simulink model "Mo_hinh_dao_chieu_dong_co_1c_kich_tu_doc_lap"  (R2016a)
settings: Solver=VariableStepAuto  StartTime=0.0  StopTime=10.0  RelTol=1e-3
libraries: powerlib x14, simulink x1
settings Model: Creator=Admin  LastModifiedBy=Admin

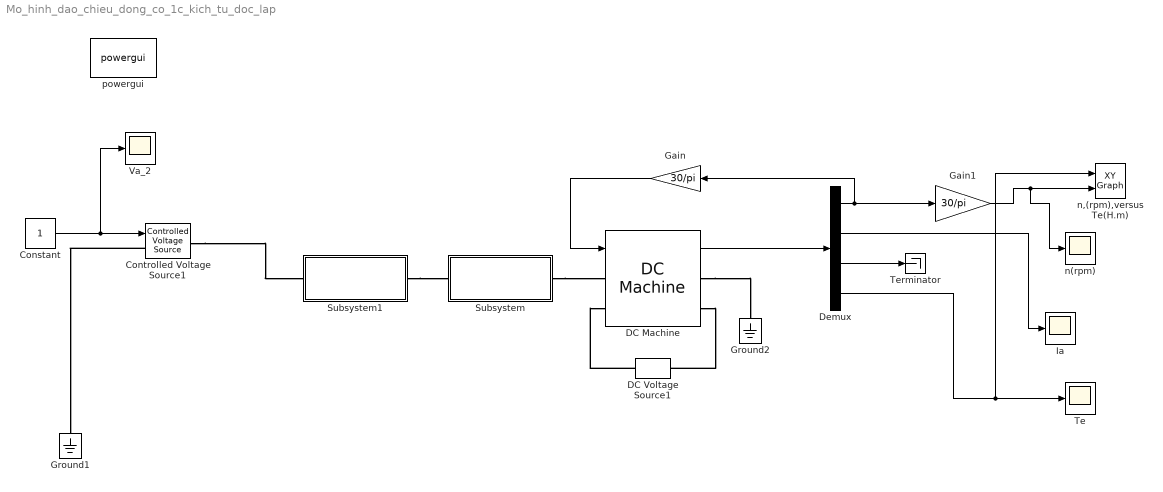
== system Mo_hinh_dao_chieu_dong_co_1c_kich_tu_doc_lap ==
  Constant : Constant
  Controlled Voltage Source1 : powerlib/Electrical Sources/Controlled Voltage Source  Initialize=on  Source_Type=AC  Amplitude=0  Phase=0  Frequency=0  Measurements=None
  DC Machine : powerlib/Machines/DC Machine  PresetModel=No  MechanicalLoad=Torque TL  FieldType=Wound  ShowDetailedParameters=on  MeasurementBus=off  RLa=[ 0.348 0.0174]  RLf=[ 0.143 0.143]  Laf=0.0174  MachineConstant=Torque constant (N.m/A)  Ke=1.8  Kt=1.8  J=1.22  Bm=0.14  Tf=2.7  w0=1  Ifinit=1  TsPowergui=0  TsBlock=-1
  DC Voltage Source1 : powerlib/Electrical Sources/DC Voltage Source  Amplitude=220  Measurements=None
  Demux : Demux
  Gain : Gain  Gain=30/pi
  Gain1 : Gain  Gain=30/pi
  Ground1 : powerlib/Elements/Ground  LConnTagsString=a
  Ground2 : powerlib/Elements/Ground  LConnTagsString=a
  "Ia " : Scope
  Subsystem : Subsystem
  Subsystem1 : Subsystem
  "Te " : Scope
  Terminator : Terminator
  "Va_2 " : Scope
  "n(rpm) " : Scope
  "n,(rpm),versus Te(H.m) " : simulink/Sinks/XY Graph  xmin=-1  xmax=1  ymin=-1  ymax=1  st=-1
  powergui : powerlib/powergui  Priority=1  SimulationMode=Continuous  SolverType=Tustin/Backward Euler (TBE)  SampleTime=50e-6  frequency=60  SPID=off  DisableSnubberDevices=off  DisableRonSwitches=off  DisableVfSwitches=off  SwTol=0  DisplayEquations=off  Interpol=off  ExternalGateDelay=off  methode=off  Ts=10  FunctionMessages=off  echomessages=off  HookPort=off  EnableUseOfTLC=off  x0status=blocks  frequencyindice=0  Pbase=100e6  ErrMax=1e-4  Iterations=50  UnitsV=kV  UnitsW=MW  buscounter=0  RestoreLinks=warning  ResistiveCurrentMeasurement=off  Frange=[0:2:500]  Ylog=off  Xlog=on  ShowGrid=off  save=off  variable=ZData  structure=0  ZoomFFT=off  StartTime=0.0  cycles=1  DisplayStyle=1  fundamental=60  FreqAxis=off  MaxFrequency=1000  frequencyindicesteady=1  RmsSteady=1  display=off
  wires:
  Gain/1 -> DC Machine/1
  DC Machine/1 -> Demux/1
  Demux/1 -> Gain1/1, Gain/1
  Demux/3 -> Terminator/1
  Gain1/1 -> "n(rpm) "/1, "n,(rpm),versus Te(H.m) "/2
  Demux/4 -> "n,(rpm),versus Te(H.m) "/1, "Te "/1
  Demux/2 -> "Ia "/1
  Constant/1 -> "Va_2 "/1, Controlled Voltage Source1/1
  connections:
  DC Machine/RConn1 -- Ground2/LConn1
  Controlled Voltage Source1/LConn1 -- Ground1/LConn1
  DC Voltage Source1/RConn1 -- DC Machine/LConn2
  DC Machine/RConn2 -- DC Voltage Source1/LConn1
  Subsystem/RConn1 -- DC Machine/LConn1
  Subsystem1/RConn1 -- Subsystem/LConn1
  Controlled Voltage Source1/RConn1 -- Subsystem1/LConn1

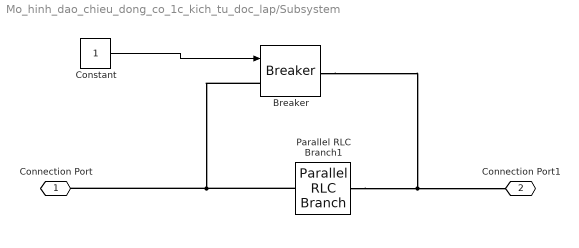
== system Mo_hinh_dao_chieu_dong_co_1c_kich_tu_doc_lap/Subsystem ==
  Breaker : powerlib/Elements/Breaker  InitialState=0  SwitchingTimes="[1/60  5/60]"  External=on  BreakerResistance=0.01  SnubberResistance=1e6  SnubberCapacitance=inf  Measurements=None  MoreParameters=on  NoBreakLoop=off
  Constant : Constant
  Parallel RLC Branch1 : powerlib/Elements/Parallel RLC Branch  LConnTagsString=a  RConnTagsString=__new0  BranchType=R  Resistance=6.04  Inductance=1e-3  SetiL0=off  InitialCurrent=0  Capacitance=1e-6  Setx0=off  InitialVoltage=0  Measurements=None
  Connection Port : PMIOPort  Port=1  Side=Left
  Connection Port1 : PMIOPort  Port=2  Side=Right
  wires:
  Constant/1 -> Breaker/1
  connections:
  Parallel RLC Branch1/RConn1 -- Breaker/LConn1 -- Connection Port/RConn1
  Parallel RLC Branch1/LConn1 -- Breaker/RConn1 -- Connection Port1/RConn1

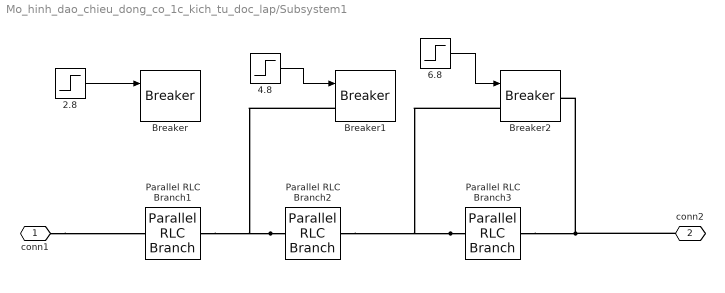
== system Mo_hinh_dao_chieu_dong_co_1c_kich_tu_doc_lap/Subsystem1 ==
  "2.8 " : Step  Time=2.8  SampleTime=0
  "4.8 " : Step  Time=4.8  SampleTime=0
  "6.8 " : Step  Time=6.8  SampleTime=0
  Breaker : powerlib/Elements/Breaker  InitialState=0  SwitchingTimes="[1/60  5/60]"  External=on  BreakerResistance=0.01  SnubberResistance=1e6  SnubberCapacitance=inf  Measurements=None  MoreParameters=on  NoBreakLoop=off
  Breaker1 : powerlib/Elements/Breaker  InitialState=0  SwitchingTimes="[1/60  5/60]"  External=on  BreakerResistance=0.01  SnubberResistance=1e6  SnubberCapacitance=inf  Measurements=None  MoreParameters=on  NoBreakLoop=off
  Breaker2 : powerlib/Elements/Breaker  InitialState=0  SwitchingTimes="[1/60  5/60]"  External=on  BreakerResistance=0.01  SnubberResistance=1e6  SnubberCapacitance=inf  Measurements=None  MoreParameters=on  NoBreakLoop=off
  Parallel RLC Branch1 : powerlib/Elements/Parallel RLC Branch  LConnTagsString=a  RConnTagsString=__new0  BranchType=R  Resistance=1  Inductance=1e-3  SetiL0=off  InitialCurrent=0  Capacitance=1e-6  Setx0=off  InitialVoltage=0  Measurements=None
  Parallel RLC Branch2 : powerlib/Elements/Parallel RLC Branch  LConnTagsString=a  RConnTagsString=__new0  BranchType=R  Resistance=1  Inductance=1e-3  SetiL0=off  InitialCurrent=0  Capacitance=1e-6  Setx0=off  InitialVoltage=0  Measurements=None
  Parallel RLC Branch3 : powerlib/Elements/Parallel RLC Branch  LConnTagsString=a  RConnTagsString=__new0  BranchType=R  Resistance=1  Inductance=1e-3  SetiL0=off  InitialCurrent=0  Capacitance=1e-6  Setx0=off  InitialVoltage=0  Measurements=None
  "conn1 " : PMIOPort  Port=1  Side=Left
  conn2 : PMIOPort  Port=2  Side=Right
  wires:
  "2.8 "/1 -> Breaker/1
  "6.8 "/1 -> Breaker2/1
  "4.8 "/1 -> Breaker1/1
  connections:
  Parallel RLC Branch3/RConn1 -- Parallel RLC Branch2/LConn1 -- Breaker2/LConn1
  Parallel RLC Branch2/RConn1 -- Parallel RLC Branch1/LConn1 -- Breaker1/LConn1
  Parallel RLC Branch3/LConn1 -- conn2/RConn1 -- Breaker2/RConn1
  "conn1 "/RConn1 -- Parallel RLC Branch1/RConn1
